simulink model "Ve"  (R2021a)
settings: Solver=VariableStepAuto  StartTime=0.0  StopTime=2474  RelTol=1e-3
undefined symbols (not defined in the file): road, tire, veh
libraries: autolibshared x1, pid_lib x1
settings Model: Creator=nileshkumark  LastModifiedBy=rahul
settings SolverCC: AlgebraicLoopSolver=TrustRegion
settings DataIOCC: ReturnWorkspaceOutputs=off
settings DebuggingCC: SFMachineParentedDataDiag=warning  ArithmeticOperatorsInVariantConditions=warning
settings SFSimCC: SimUseLocalCustomCode=off  CustomCodeUndefinedFunction=UseInterfaceOnly
settings RTWCC: RTWUseLocalCustomCode=off

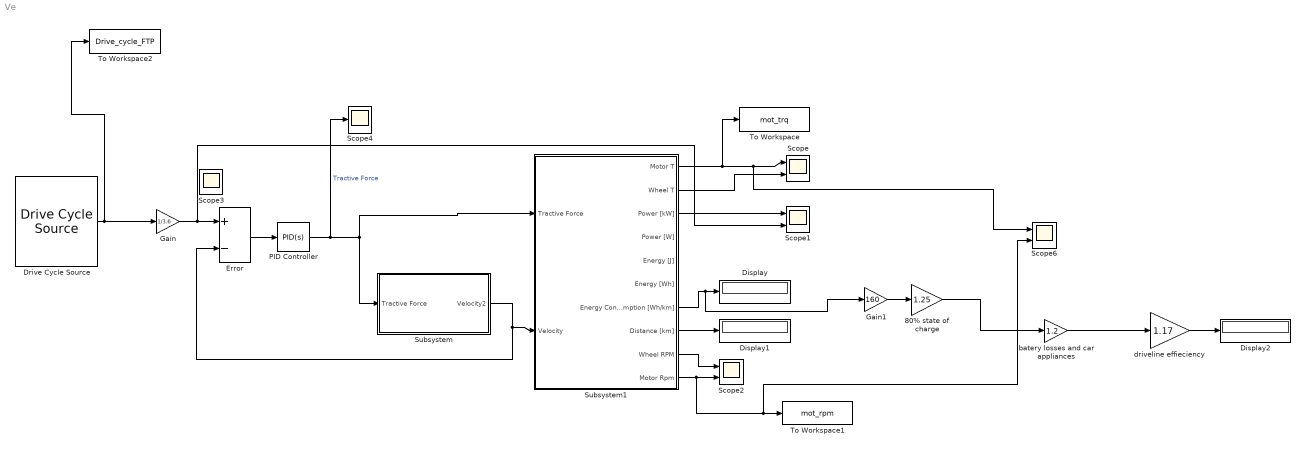
== system Ve ==
  80% state of charge : Gain  Gain=1.25
  Display : Display
  Display1 : Display
  Display2 : Display
  Drive Cycle Source : autolibshared/Drive Cycle Source  cycleVar=FTP75  fileVar=cycleFTP75.mat  tfinal="2474  seconds"  cycleRepeat=off  outAccPort=off  outGearPort=off  gearList=No gear data  t_wot1=5  xdot_woto=0  xdot_wot1=30  t_wot2=20  xdot_wot2=0  t_wotend=30  srcUnit=m/s  outUnit=km/h  srcAccUnit=m/s/s  outAccUnit=m/s^2  dt=0  aMode=1  faultOption=off  velBnd=2  velBndUnit=mph  inUnit=m/s  timeBnd=1  failOption=off  stopSim=off  maxFaultCnt=10  maxFaultTime=2  maxTotFaultTime=15  traceOption=off  dtTrace=1  traceWindow=10  lastDCname=FTP75  lastOutUnit=mph  lastDT=0  lastTB=1  lastSB=2  forceCalcBound=off
      settings: SourceProductBaseCode=PW,DR,MT,UV,VE
  Error : Sum  Inputs=+-
  Gain : Gain  Gain=1/3.6
  Gain1 : Gain  Gain=160
  PID Controller : pid_lib/PID Controller  Controller=PID  Form=Parallel  TimeDomain=Continuous-time  UseExternalTs=off  SampleTime=-1  IntegratorMethod=Forward Euler  FilterMethod=Forward Euler  ControllerParametersSource=internal  P=900  I=0.001  D=0  UseFilter=on  N=100  TunerSelectOption=Transfer Function Based (PID Tuner App)  InitialConditionSource=internal  InitialConditionForIntegrator=0  InitialConditionForFilter=0  DifferentiatorICPrevScaledInput=0  ExternalReset=none  TrackingMode=off  Kt=1  LimitOutput=off  SatLimitsSource=internal  UpperSaturationLimit=inf  LowerSaturationLimit=-inf  LinearizeAsGain=on  AntiWindupMode=none  Kb=1  POutMin=[]  POutMax=[]  IOutMin=[]  IOutMax=[]  DOutMin=[]  DOutMax=[]  NOutMin=[]  NOutMax=[]  SumOutMin=[]  SumOutMax=[]  SaturationOutMin=[]  SaturationOutMax=[]  PParamMin=[]  PParamMax=[]  IParamMin=[]  IParamMax=[]  DParamMin=[]  DParamMax=[]  NParamMin=[]  NParamMax=[]  KbParamMin=[]  KbParamMax=[]  KtParamMin=[]  KtParamMax=[]  KbOutMin=[]  KbOutMax=[]  KtOutMin=[]  KtOutMax=[]  IntegratorOutMin=[]  IntegratorOutMax=[]  FilterOutMin=[]  FilterOutMax=[]  SumI1OutMin=[]  SumI1OutMax=[]  SumI2OutMin=[]  SumI2OutMax=[]  SumI3OutMin=[]  SumI3OutMax=[]  SumI4OutMin=[]  SumI4OutMax=[]  SumDOutMin=[]  SumDOutMax=[]  DifferentiatorOutMin=[]  DifferentiatorOutMax=[]  FilterDiffOutCoefMin=[]  FilterDiffOutCoefMax=[]  ReciprocalOutMin=[]  ReciprocalOutMax=[]  SumDenOutMin=[]  SumDenOutMax=[]  SumNumOutMin=[]  SumNumOutMax=[]  DivideOutMin=[]  DivideOutMax=[]  UdiffTsProdOutMin=[]  UdiffTsProdOutMax=[]  NTsProdOutMin=[]  NTsProdOutMax=[]  UintegralTsProdOutMin=[]  UintegralTsProdOutMax=[]  UngainTsProdOutMin=[]  UngainTsProdOutMax=[]  IntegratorContinuousStateAttributes=''  IntegratorStateMustResolveToSignalObject=off  IntegratorRTWStateStorageClass=Auto  FilterContinuousStateAttributes=''  FilterStateMustResolveToSignalObject=off  FilterRTWStateStorageClass=Auto  ParallelPVariant=InternalParameters  IdealPVariant=Disabled  IVariant=InternalParameters  DVariant=InternalParameters  IntegratorVariant=Continuous  SatVariant=Disabled  AWVariant=Passthrough  PCopyVariant=Disabled  TRVariant=Disabled  FdbkBlocksVariant=Forward  IdealPFdbkVariant=Disabled  SatFdbkVariant=Disabled  DerivativeFilterVariant=ContFilter  NVariant=InternalParameters  NCopyVariant=Disabled  FilterICVariant=InternalICsFilter  IntegratorICVariant=InternalICs  ExternalResetVariant=Disabled  TRSumVariant=Passthrough  SumFdbkVariant=Disabled  SumVariant=Sum_PID  TsampFilterVariant=InternalTs  TsampNgainVariant=Passthrough  TsampIntegralVariant=Passthrough  ExternalSaturationOutDataTypeStr=Inherit: Same as second input
  Scope{,1..2,6} (4 alike) : Scope  NumInputPorts=2
  Scope4 : Scope
  Subsystem : Subsystem
  Subsystem1 : Subsystem
  To Workspace : ToWorkspace  VariableName=mot_trq  SampleTime=1
  To Workspace1 : ToWorkspace  VariableName=mot_rpm  SampleTime=1
  To Workspace2 : ToWorkspace  VariableName=Drive_cycle_FTP  SaveFormat=Structure With Time  SampleTime=-1
  batery losses and car appliances : Gain  Gain=1.2
  driveline effieciency : Gain  Gain=1.17
  Scope3 : Scope
  wires:
  PID Controller/1 -> Scope4/1, Subsystem1/1(Tractive Force), Subsystem/1(Tractive Force)  "Tractive Force"
  Subsystem/1(Velocity2) -> Subsystem1/2(Velocity), Error/2
  Drive Cycle Source/1 -> To Workspace2/1, Gain/1
  Gain/1 -> Scope1/2, Error/1
  Error/1 -> PID Controller/1
  Subsystem1/1(Motor T) -> To Workspace/1, Scope6/1, Scope/1
  Subsystem1/3(Power [kW]) -> Scope1/1
  Subsystem1/7(Energy Consumption [Wh/km]) -> Gain1/1, Display/1
  Subsystem1/8(Distance [km]) -> Display1/1
  Subsystem1/10(Motor Rpm) -> Scope6/2, To Workspace1/1, Scope2/2
  Subsystem1/9(Wheel RPM) -> Scope2/1
  Subsystem1/2(Wheel T) -> Scope/2
  Gain1/1 -> 80% state of charge/1
  80% state of charge/1 -> batery losses and car appliances/1
  batery losses and car appliances/1 -> driveline effieciency/1
  driveline effieciency/1 -> Display2/1

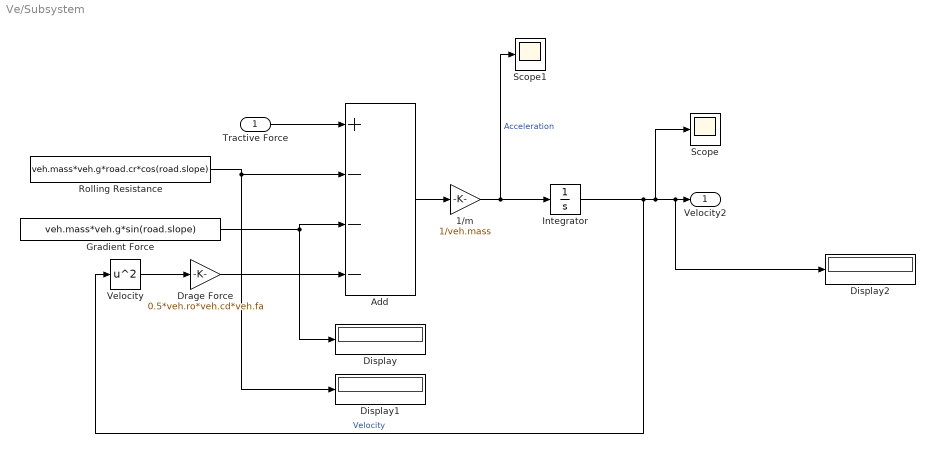
== system Ve/Subsystem ==
  Tractive Force : Inport
  1/m : Gain  Gain=1/veh.mass
  Add : Sum  Inputs=+---
  Display : Display
  Display1 : Display
  Display2 : Display
  Drage Force : Gain  Gain=0.5*veh.ro*veh.cd*veh.fa
  Gradient Force : Constant  Value=veh.mass*veh.g*sin(road.slope)
  Integrator : Integrator
  Rolling Resistance : Constant  Value=veh.mass*veh.g*road.cr*cos(road.slope)
  Scope : Scope
  Scope1 : Scope
  Velocity : Math  Operator=square  SignedPower=on  SaturateOnIntegerOverflow=on
  Velocity2 : Outport  VectorParamsAs1DForOutWhenUnconnected=off
  wires:
  Add/1 -> 1/m/1
  Drage Force/1 -> Add/4
  1/m/1 -> Scope1/1, Integrator/1  "Acceleration"
  Rolling Resistance/1 -> Display1/1, Add/2
  Tractive Force/1 -> Add/1
  Velocity/1 -> Drage Force/1
  Gradient Force/1 -> Add/3, Display/1
  Integrator/1 -> Velocity/1, Scope/1, Display2/1, Velocity2/1  "Velocity"

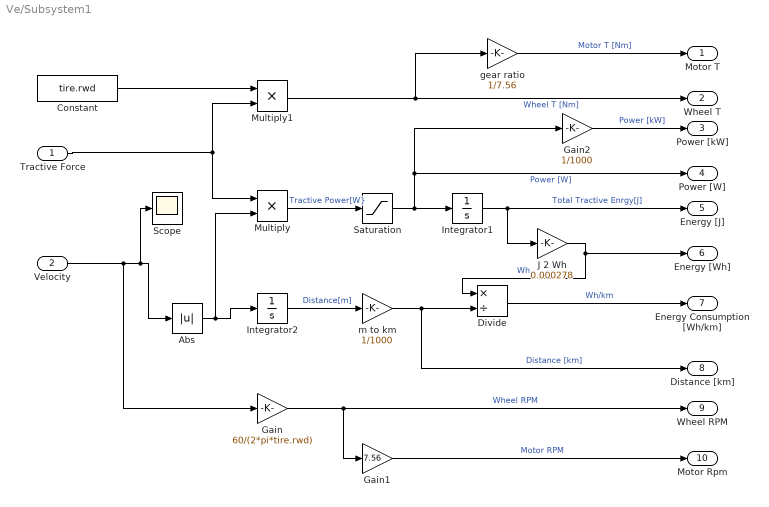
== system Ve/Subsystem1 ==
  Tractive Force : Inport
  Velocity : Inport  Port=2
  Abs : Abs
  Constant : Constant  Value=tire.rwd
  Divide : Product  Inputs=*/
  Gain : Gain  Gain=60/(2*pi*tire.rwd)
  Gain1 : Gain  Gain=7.56
  Gain2 : Gain  Gain=1/1000
  Integrator1 : Integrator
  Integrator2 : Integrator
  J 2 Wh : Gain  Gain=0.000278
  Multiply : Product
  Multiply1 : Product
  Saturation : Saturate  UpperLimit=inf  LowerLimit=0
  Scope : Scope
  gear ratio : Gain  Gain=1/7.56
  m to km : Gain  Gain=1/1000
  Motor T : Outport  VectorParamsAs1DForOutWhenUnconnected=off
  Wheel T : Outport  Port=2  VectorParamsAs1DForOutWhenUnconnected=off
  Power [kW] : Outport  Port=3  VectorParamsAs1DForOutWhenUnconnected=off
  Power [W] : Outport  Port=4  VectorParamsAs1DForOutWhenUnconnected=off
  Energy [J] : Outport  Port=5  VectorParamsAs1DForOutWhenUnconnected=off
  Energy [Wh] : Outport  Port=6  VectorParamsAs1DForOutWhenUnconnected=off
  Energy Consumption [Wh/km] : Outport  Port=7  VectorParamsAs1DForOutWhenUnconnected=off
  Distance [km] : Outport  Port=8  VectorParamsAs1DForOutWhenUnconnected=off
  Wheel RPM : Outport  Port=9  VectorParamsAs1DForOutWhenUnconnected=off
  Motor Rpm : Outport  Port=10  VectorParamsAs1DForOutWhenUnconnected=off
  wires:
  Tractive Force/1 -> Multiply/1, Multiply1/2
  m to km/1 -> Distance [km]/1, Divide/2  "Distance [km]"
  Integrator1/1 -> Energy [J]/1, J 2 Wh/1  "Total Tractive Enrgy[J]"
  Multiply/1 -> Saturation/1  "Tractive Power[W}"
  Divide/1 -> Energy Consumption [Wh/km]/1  "Wh/km"
  Integrator2/1 -> m to km/1  "Distance[m]"
  J 2 Wh/1 -> Energy [Wh]/1, Divide/1  "Wh"
  Saturation/1 -> Power [W]/1, Gain2/1, Integrator1/1  "Power [W]"
  Constant/1 -> Multiply1/1
  Multiply1/1 -> Wheel T/1, gear ratio/1  "Wheel T [Nm]"
  gear ratio/1 -> Motor T/1  "Motor T [Nm]"
  Gain/1 -> Gain1/1, Wheel RPM/1  "Wheel RPM"
  Gain1/1 -> Motor Rpm/1  "Motor RPM"
  Gain2/1 -> Power [kW]/1  "Power [kW]"
  Velocity/1 -> Gain/1, Scope/1, Abs/1
  Abs/1 -> Multiply/2, Integrator2/1
